simulink model "llc_resonant_converter"  (Simulink 7.3)
settings: Solver=ode45  StartTime=0.0  StopTime=Tend  MaxStep=1e-3  RelTol=1e-4
InitFcn:
  | %% Processor selection for I/O assignment
  | %% The chosen Target in the Coder Options window must match the selected MCU.
  | %% Set the variable 'type_evm' to the following strings to choose a specific target:
  | 
  | % type_evm = 'TI28377S';                  % TI28377S Delfino Launchpad
  |   type_evm = 'TI28379LP';                   % TI28379D Delfino Launchpad
  | % type_evm = 'TI28379CC';                % TI28379D Delfino Controlcard
  | % type_evm = 'TI28388D';                  % TI28388D Controlcard
  | 
  | %% Time-scaling settings.
  | scale = 0.1;					% Time-scaling factor.  Less than 1 is slower than real-time.
  | Ts_plant = 0.40e-6/scale;	% Plant discretization as Ts_plant_unscaled/scale. Ts_plant_unscaled can be less than 1us with appropriate scaling factor.
  | 
  | %% TI Evaluation Board parameters
  | Lm = 280e-6/scale;                              % Magnetizing inductance
  | Ls = 55e-6/scale;                                 % Series resonant inductance
  | Cs = 24e-9/scale;                                 % Series resonant capacitance
  | Cf = 1.33e-3/scale;                               % Output capcitance
  | rd = 0.00725 + 0.01;                           % Secondary MOSFET and secondary side lump resistance
  | rc = 1.33e-3;                                       % Output filter capacitor ESR
  | rs = 15e-3;                                          % Series resiatance of resonance inductor
  | n = 17;                                                % Transformer turns ration - Np/Ns
  | 
  | %% LLC Operating Point
  | Duty = 0.5;                                          % Duty ratio
  | Vin = 390;                                           % Input voltage
  | Po_desired = 300;                               % Output power
  | Vo = 12;                                              % Output voltage
  | Io = Po_desired/Vo;                             % Output current
  | R = Vo/Io;                                           % Load resistance
  | Re = (8*(n^2)/(pi^2))*(rd+R);            % AC equivalent secondary resistance refer to primary
  | 
  | fsw = 110e3*scale;                              % Nominal switching frequency for PWM (Variable) and control
  | Ts = 2/(fsw);                                       % Sampling time
  | Tload_period = 0.04/scale;                   % Period for load resistance toggling
  | Tend = 0.05/scale;                               % Simulation duration
  | 
  | %% Finding switching frequency based on Gain-Frequency Curve
  | Vq = (Vin/2);                                       % Half-bridge voltage
  | 
  | W0 = 1/sqrt(Ls*Cs) ;                            % Resonance frequency in Rad/s
  | f0 = W0/(2*pi);                                    % Resonance frequency in Hz
  | 
  | m = (Lm+Ls)/Ls;                                  % LLC inductance ratio
  | Qfac = sqrt(Ls/Cs)/Re;                          % Q-factor of LLC tank circuit for specific load resistance
  | GainR = n*(Vo+(rd*Io))/Vq;                 % Required resonance tank gain
  | 
  | %% Finding ratio of switching frequency to resonance frequency
  | Aa = (Qfac^2)*((m-1)^2);
  | Bb = (m^2)-(2*(Qfac^2)*((m-1)^2))-(((m-1)^2)/(GainR^2));
  | Cc = ((Qfac^2)*((m-1)^2))-(2*m);
  | Dd = 1;
  | Fxp = [Aa 0 Bb 0 Cc 0 Dd];
  | Fxr = roots(Fxp);
  | Fxreal = real(Fxr);
  | Fx = max(Fxreal);                                % Ratio of switching frequency to resonance frequency
  | fs = Fx*f0;                                           % Switching frequency related to load resistance
  | 
  | %% 2P2Z Controller Parameters calculated using EDF and pole-zero matching
  | Gcv_d_den = [1 -0.325769999305 -0.674230000695];
  | Gcv_d_num = [0.2365162756 -0.277992922163 0.0988826256903];
  | 
  | %% Soft-start settings
  | Tduty_ramp = 0.005/scale;
  | Tfreq_ramp = 0.005/scale;
  | Duty_init = 0;
  | Duty_final=0.5;
  | Freq_init = 1.5*Fx;
  | Freq_final = Fx;
  | 
  | %% Controller discretization configuration
  | Ts_controller = Ts;			          % Automatically calculated and scaled.
  | 
  | %% Configure I/O based on processor
  | switch (type_evm)
  | 	case 'TI28377S'
  | 	% Configuration for TI28377S Launchpad
  | 		% On the Plant side
  | 		AO_RTBox_Vo = 12;
  | 		PWMCAP_RTBox_sw = [20:21];
  | 		DI_RTBox_Eni = 29;
  | 		DO_RTBox_Eno = 6;
  | 		DI_RTBox_Power = 26;
  | 		AO_Vmax = 3.3;
  | 		AO_Factor = 1;
  | 
  | 		% On the Controller side
  | 		ADC_DSP_ADC = 3;
  | 		PWM_DSP_PWM = 4; %PWM Group - 1=ePWM1, 2=ePWM4, 3=ePWM7, 4=ePWM10
  | 		DO_DSP_LED = 12;
  | 		DI_DSP_En = 72;
  | 		PWR_DSP_GPIO = 43;
  | 		SCI_DSP = [85,84];
  | 		ADC_Vmax = 3.3;
  | 
  | 
  | 	case 'TI28379LP'
  | 	% Configuration for TI28379D Launchpad
  | 		% On the Plant side
  | 		AO_RTBox_Vo = 14;
  | 		PWMCAP_RTBox_sw = [0:1];
  | 		DI_RTBox_Eni = 29;
  | 		DO_RTBox_Eno = 6;
  | 		DI_RTBox_Power = 22;
  | 		AO_Vmax = 3.3;
  | 		AO_Factor = 1;
  | 
  | 		% On the Controller side
  | 		ADC_DSP_ADC = 4;
  | 		PWM_DSP_PWM = 1; %PWM Group - 1=ePWM1, 2=ePWM4, 3=ePWM7, 4=ePWM10
  | 		DO_DSP_LED = 34;
  | 		DI_DSP_En = 124;
  | 		PWR_DSP_GPIO = 66;
  | 		SCI_DSP = [43, 42];
  | 		ADC_Vmax = 3.3;
  | 
  | 	case 'TI28379CC'
  | 	% Configuration for TI28379D Controlcard
  | 	   % On the Plant side
  | 		AO_RTBox_Vo = 15;
  | 		PWMCAP_RTBox_sw = 0:1;
  | 		DI_RTBox_Eni = 29;
  | 		DO_RTBox_Eno = 21;
  | 		DI_RTBox_Power = 14;
  | 		AO_Vmax = 5.0;
  | 		AO_Factor = 1.54; % breakout board scaling 6.8k/4.42k
  | 
  | 		% On the Controller side
  | 		ADC_DSP_ADC = 0;
  | 		PWM_DSP_PWM = 1;
  | 		DO_DSP_LED = 34;
  | 		DI_DSP_En = 40;
  | 		PWR_DSP_GPIO = 39;
  | 		SCI_DSP = [28, 29];
  | 		ADC_Vmax = 3.0;
  | 
  | 	case 'TI28388D'
  | 	% Configuration for TI28388D Controlcard
  | 	  % On the Plant side
  | 		AO_RTBox_Vo = 15;
  | 		PWMCAP_RTBox_sw = 0:1;
  | 		DI_RTBox_Eni = 29;
  | 		DO_RTBox_Eno = 21;
  | 		DI_RTBox_Power = 14;
  | 		AO_Vmax = 5.0;
  | 		AO_Factor = 1.54; % breakout board scaling 6.8k/4.42k
  | 
  | 		% On the Controller side
  | 		ADC_DSP_ADC = 0;
  | 		PWM_DSP_PWM = 1;
  | 		DO_DSP_LED = 34;
  | 		DI_DSP_En = 40;
  | 		PWR_DSP_GPIO = 39;
  | 		SCI_DSP = [28, 29];
  | 		ADC_Vmax = 3.0;
  | 
  | 	otherwise
  | 	error('Unknown evaluation module selection, please choose either ''TI28377S'', ''TI28379LP'', ''TI28335'', ''TI28379CC'' or ''TI28388D''.')
  | end
  | 
  | 
  | %% RT Box analog IO scaling
  | Vo_scl = ADC_Vmax/Vo/2;
  | 
  | %% Remove complex variables from workspace.
  | clear('Fxr')
undefined symbols (not defined in the file): plecs
settings Model: Creator=kris  LastModifiedBy=manaswini  ExtModeTrigMode=oneshot  ExtModeArmWhenConnect=off  ExtModeAutoUpdateStatusClock=off
settings DataIOCC: LimitDataPoints=off  ReturnWorkspaceOutputs=off  SignalLoggingName=sigsOut
settings OptimizationCC: BooleanDataType=off  ExpressionDepthLimit=128  InitFltsAndDblsToZero=on
settings DebuggingCC: SaveWithParameterizedLinksMsg=none  SignalResolutionControl=TryResolveAllWithWarning  SolverPrmCheckMsg=none  MultiTaskDSMMsg=warning  MultiTaskCondExecSysMsg=none  FcnCallInpInsideContextMsg=Enable All  StrictBusMsg=ErrorLevel1
settings HardwareCC: TargetHWDeviceType=32-bit Generic  TargetUnknown=on  ProdEqTarget=off
settings RTWCC: IncludeERTFirstTime=on
settings CodeAppCC: CustomSymbolStrType=$N$R$M_T
settings GRTTargetCC: TargetFcnLib=ansi_tfl_tmw.mat  TargetFunctionLibrary=C89/C90 (ANSI)  ModelReferenceCompliant=off

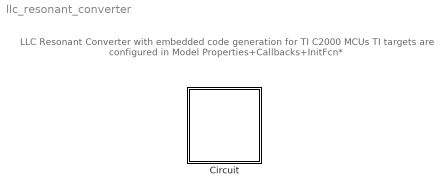
== system llc_resonant_converter ==
  note: LLC Resonant Converter
      | with embedded code generation for TI C2000 MCUs
      | TI targets are configured in Model Properties+Callbacks+InitFcn*
  Circuit : Subsystem  LoadFcn=plecs('sl', 200);  InitFcn=plecs('sl', 214);  StartFcn=plecs('sl', 208);  StopFcn=plecs('sl', 209);  ClipboardFcn=plecs('sl', 212, 28);  mask(PlecsCircuit){PLECSData=<binary blob, 21420 chars, not shown>}
      mask prompts: PLECSData "PLECS Data (Do not delete or modify!)"
      mask help: Drag this block into a Simulink model to create a new electrical circuit.
      mask init:
      | % PLACE CUSTOM INITIALIZATIONS ABOVE
      | % DO NOT REMOVE
      | plecs('sl', 215);
      | % DO NOT REMOVE
      settings: CopyFcn=plecs('sl', 203);  DeleteFcn=plecs('sl', 205);  UndoDeleteFcn=plecs('sl', 206);  PreSaveFcn=plecs('sl', 211);  PostSaveFcn=plecs('sl', 201);  NameChangeFcn=plecs('sl', 210);  DestroyFcn=plecs('sl', 207);  PreCopyFcn=plecs('sl', 216);  OpenFcn=plecs('sl', 202);  ErrorFcn=plerrorfcn
      mask Display: disp('PLECS\nCircuit')

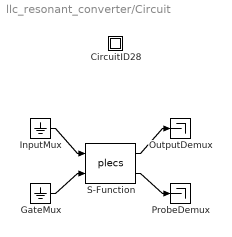
== system llc_resonant_converter/Circuit ==
  " CircuitID28 " : Subsystem
  " GateMux " : Ground
  " InputMux " : Ground
  " OutputDemux " : Terminator
  " ProbeDemux " : Terminator
  " S-Function " : S-Function  FunctionName=plecs  EnableBusSupport=off
  wires:
  " InputMux "/1 -> " S-Function "/1
  " GateMux "/1 -> " S-Function "/2
  " S-Function "/1 -> " OutputDemux "/1
  " S-Function "/2 -> " ProbeDemux "/1

== system llc_resonant_converter/Circuit/ CircuitID28  ==
